simulink model "untitled"  (R2020b)
settings: Solver=VariableStepAuto  StartTime=0.0  StopTime=10.0  RelTol=1e-3
settings Model: Creator=sai  LastModifiedBy=sai

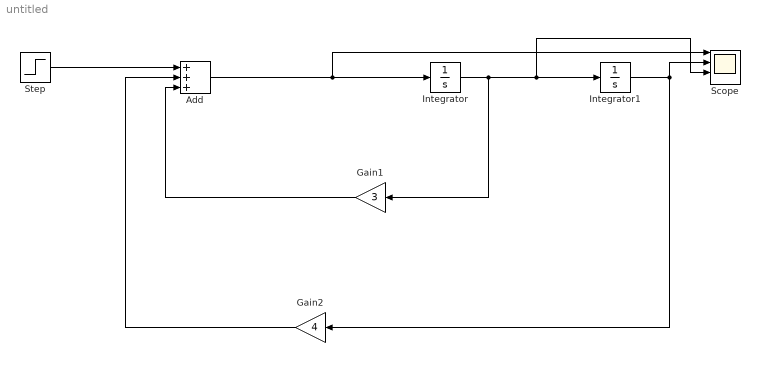
== system untitled ==
  Add : Sum  Inputs=+++
  Gain1 : Gain  Gain=3
  Gain2 : Gain  Gain=4
  Integrator : Integrator
  Integrator1 : Integrator
  Scope : Scope  NumInputPorts=4
  Step : Step  Time=5  SampleTime=0
  wires:
  Step/1 -> Add/1
  Gain2/1 -> Add/2
  Gain1/1 -> Add/3
  Integrator/1 -> Gain1/1, Scope/3, Integrator1/1
  Integrator1/1 -> Scope/2, Gain2/1
  Add/1 -> Scope/1, Integrator/1
